simulink model "practica1_ariel"  (R2023b)
settings: Solver=VariableStepAuto  StartTime=0.0  StopTime=18  RelTol=1e-3
undefined symbols (not defined in the file or in its folder): DiscIntNeverNeededParam, Gz
libraries: SignalEditorBlockLib x1
settings Model: Creator=Usuario_UMA  LastModifiedBy=Usuario_UMA

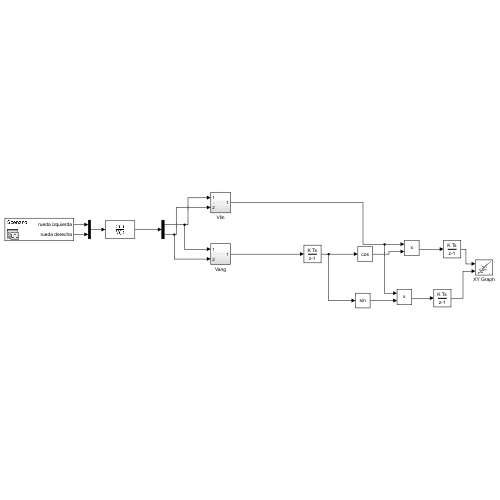
[thumbnail: Simulink's stored preview of the top-level diagram]
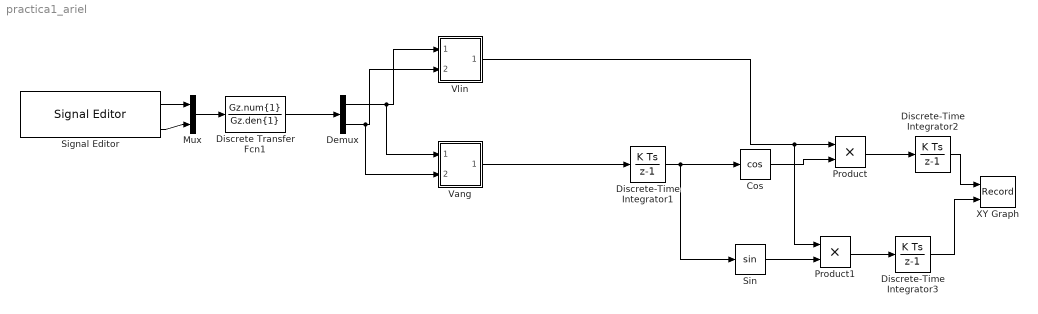
== system practica1_ariel ==
  Cos : Trigonometry  Operator=cos
  Demux : Demux  Outputs=2
  Discrete Transfer Fcn1 : DiscreteTransferFcn  Numerator=Gz.num{1}  Denominator=Gz.den{1}
  Discrete-Time Integrator1 : DiscreteIntegrator  SampleTime=0.025  ICPrevOutput=DiscIntNeverNeededParam  ICPrevScaledInput=DiscIntNeverNeededParam
  Discrete-Time Integrator2 : DiscreteIntegrator  SampleTime=0.025  ICPrevOutput=DiscIntNeverNeededParam  ICPrevScaledInput=DiscIntNeverNeededParam
  Discrete-Time Integrator3 : DiscreteIntegrator  SampleTime=0.025  ICPrevOutput=DiscIntNeverNeededParam  ICPrevScaledInput=DiscIntNeverNeededParam
  Mux : Mux  Inputs=2
  Product : Product
  Product1 : Product
  Signal Editor : SignalEditorBlockLib/Signal Editor  FileName=C:\Users\Usuario_UMA\Downloads\signaleditor_p1.mat  ActiveScenario=Scenario  ActiveSignal=rueda izquierda  IsBus=off  OutputBusObjectStr=Bus: BusObject  SampleTime=0  Interpolate=off  ZeroCross=off  OutputAfterFinalValue=Setting to zero  Unit=inherit  PreserveSignalName=on  ApplySigPropsToAllScenarios=on  ApplySigPropsToAllSignals=off
  Sin : Trigonometry
  Vang : Subsystem
  Vlin : Subsystem
  XY Graph : Record  FileSettingsInternal="{\"entries\":[{\"content\":{\"excelSettings\":{\"content\":{},\"type\":\"Streamout.ExcelSettings\"}},\"type\":\"Streamout.FileSettingStorage\",\"uuid\":\"\"}],\"packageUris\":[\"http:\\/\\/schema.mathworks.com\\/mf0\\/streamout_blocks\\/R2020a\"],\"version\":\"1.0\"}"  Layout=[1 1]  SignalsInternal="{\"entries\":[{\"content\":{\"signals\":[{\"content\":{\"blockPath\":[],\"dimensions\":[1],\"domain\":\"\",\"lineColor\":\"#ff6929\",\"plots\":[1],\"port\":1,\"sid\":[\"\"],\"signalID\":356,\"signalName\":\"Discrete-Time\\nIntegrator2\"},\"type\":\"RecordBlkView.Signal\",\"uuid\":\"\"},{\"content\":{\"blockPath\":[],\"dimensions\":[1],\"domain\":\"\",\"lineColor\":\"#b746ff\",\"plots\":[1],\"port\":2,\"sid\":[\"\"],\"signalID\":360,\"signalName\":\"Discrete-Time\\nIntegrator3\"},\"type\":\"RecordBlkView.Signal\",\"uuid\":\"\"}]},\"type\":\"RecordBlkView.InputSignals\",\"uuid\":\"\"}],\"packageUris\":[\"http:\\/\\/schema.mathworks.com\\/mf0\\/streamout_blocks\\/R2020a\"],\"version\":\"1.0\"}"  VisualizationBindings="{\"xyplotplugin\":{\"info\":[{\"series\":[{\"bindingParametersList\":[{\"parameter\":\"X-Axis\",\"signalID\":356,\"signalName\":\"Discrete-Time\\nIntegrator2\"},{\"parameter\":\"Y-Axis\",\"signalID\":360,\"signalName\":\"Discrete-Time\\nIntegrator3\"}],\"seriesID\":61526}],\"subplotID\":1}]}}"  CompatibilityTag=XY
  wires:
  Discrete-Time Integrator1/1 -> Sin/1, Cos/1
  Cos/1 -> Product/2
  Vang/1(Out1) -> Discrete-Time Integrator1/1
  Vlin/1(Out1) -> Product1/1, Product/1
  Product/1 -> Discrete-Time Integrator2/1
  Discrete-Time Integrator2/1 -> XY Graph/1
  Sin/1 -> Product1/2
  Product1/1 -> Discrete-Time Integrator3/1
  Discrete-Time Integrator3/1 -> XY Graph/2
  Mux/1 -> Discrete Transfer Fcn1/1
  Demux/1 -> Vang/1(In1), Vlin/1(In1)
  Demux/2 -> Vang/2(In2), Vlin/2(In2)
  Discrete Transfer Fcn1/1 -> Demux/1
  Signal Editor/1 -> Mux/1
  Signal Editor/2 -> Mux/2

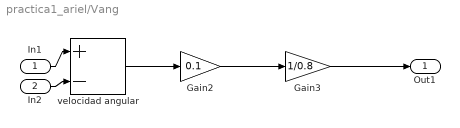
== system practica1_ariel/Vang ==
  In1 : Inport
  In2 : Inport  Port=2
  Gain2 : Gain  Gain=0.1
  Gain3 : Gain  Gain=1/0.8
  velocidad angular : Sum  Inputs=|+-
  Out1 : Outport
  wires:
  Gain3/1 -> Out1/1
  velocidad angular/1 -> Gain2/1
  Gain2/1 -> Gain3/1
  In2/1 -> velocidad angular/2
  In1/1 -> velocidad angular/1

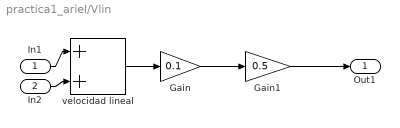
== system practica1_ariel/Vlin ==
  In1 : Inport
  In2 : Inport  Port=2
  Gain : Gain  Gain=0.1
  Gain1 : Gain  Gain=0.5
  velocidad lineal : Sum  Inputs=|++
  Out1 : Outport
  wires:
  In1/1 -> velocidad lineal/1
  Gain1/1 -> Out1/1
  Gain/1 -> Gain1/1
  velocidad lineal/1 -> Gain/1
  In2/1 -> velocidad lineal/2
